simulink model "adaptiveObs"  (R2012b)
settings: Solver=ode45  StartTime=0.0  StopTime=TStop  MaxStep=Ts  RelTol=10e-5
values from neighbouring files (symbols this model uses):
  A = [-5 1; -10 0]    [adaptiveObsRun.m]
  a1hat0 = 3    [adaptiveObsRun.m]
  a2hat0 = 12    [adaptiveObsRun.m]
  B = [1;2]    [adaptiveObsRun.m]
  b1hat0 = 0.5    [adaptiveObsRun.m]
  b2hat0 = 1    [adaptiveObsRun.m]
  C = [1 0]    [adaptiveObsRun.m]
settings Model: Creator=sqn4594  LastModifiedBy=sqn4594
settings SolverCC: AlgebraicLoopSolver=LineSearch
settings DataIOCC: SignalLoggingSaveFormat=ModelDataLogs
settings DebuggingCC: MultiTaskDSMMsg=warning  MultiTaskCondExecSysMsg=none  StrictBusMsg=None
settings RTWCC: IncludeERTFirstTime=on
settings CodeAppCC: CustomSymbolStrType=$N$R$M_T  InternalIdentifier=Shortened

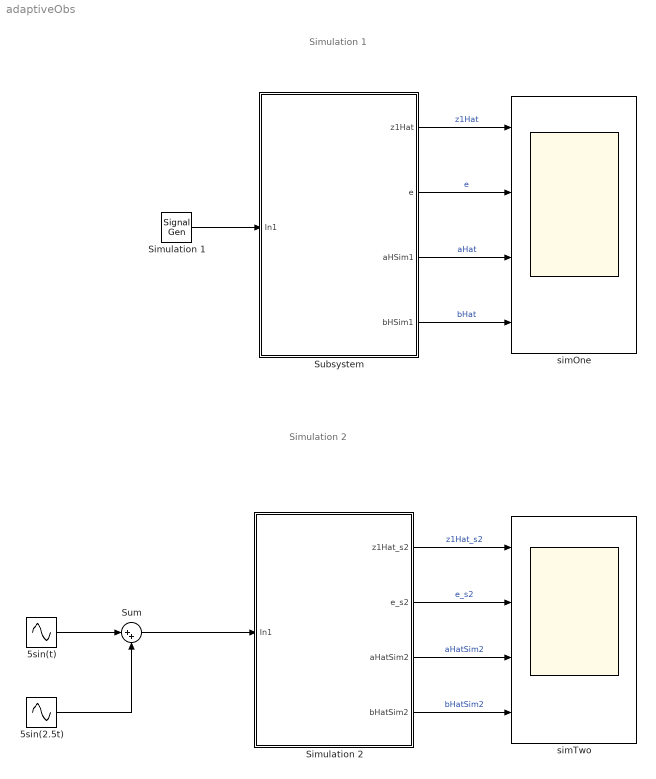
== system adaptiveObs ==
  note: Simulation 1
  note: Simulation 2
  5sin(2.5t) : Sin  Amplitude=5  Frequency=2.5  SampleTime=0
  5sin(t) : Sin  Amplitude=5  SampleTime=0
  Simulation 1 : SignalGenerator  WaveForm=square  Amplitude=5  Units=rad/sec
  Simulation 2 : Subsystem
  Subsystem : Subsystem
  Sum : Sum  Inputs=|++
  "simOne " : Scope  NumInputPorts=4
      settings: YMin=-5~-5~-5~-5  YMax=5~5~5~5  SaveName=simOne
  simTwo : Scope  NumInputPorts=4
      settings: YMin=-5~-5~-5~-5  YMax=5~5~5~5  SaveName=simTwo
  wires:
  5sin(t)/1 -> Sum/1
  5sin(2.5t)/1 -> Sum/2
  Simulation 1/1 -> Subsystem/1(In1)
  Sum/1 -> Simulation 2/1(In1)
  Subsystem/1(z1Hat) -> "simOne "/1  "z1Hat"
  Subsystem/2(e) -> "simOne "/2  "e"
  Subsystem/3(aHSim1) -> "simOne "/3  "aHat"
  Subsystem/4(bHSim1) -> "simOne "/4  "bHat"
  Simulation 2/1(z1Hat_s2) -> simTwo/1  "z1Hat_s2"
  Simulation 2/2(e_s2) -> simTwo/2  "e_s2"
  Simulation 2/3(aHatSim2) -> simTwo/3  "aHatSim2"
  Simulation 2/4(bHatSim2) -> simTwo/4  "bHatSim2"

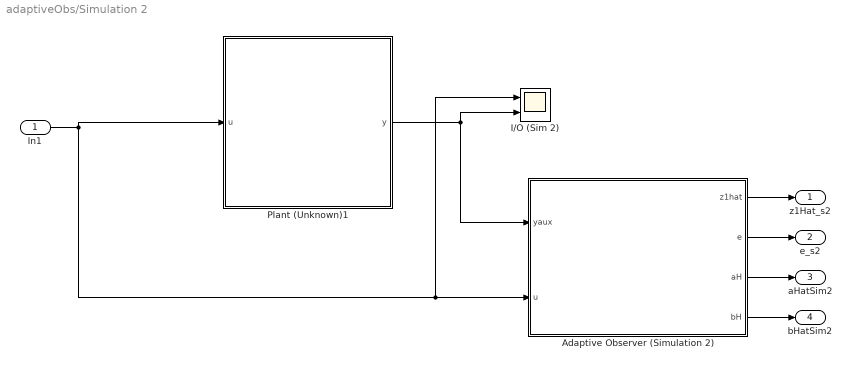
== system adaptiveObs/Simulation 2 ==
  In1 : Inport
  Adaptive Observer (Simulation 2) : Subsystem
  I/O (Sim 2) : Scope  NumInputPorts=2
      settings: YMin=-5~-5  YMax=5~5  SaveName=uy1
  Plant (Unknown)1 : Subsystem
  z1Hat_s2 : Outport
  e_s2 : Outport  Port=2
  aHatSim2 : Outport  Port=3
  bHatSim2 : Outport  Port=4
  wires:
  In1/1 -> Plant (Unknown)1/1(u), Adaptive Observer (Simulation 2)/2(u), I/O (Sim 2)/1
  Plant (Unknown)1/1(y) -> I/O (Sim 2)/2, Adaptive Observer (Simulation 2)/1(yaux)
  Adaptive Observer (Simulation 2)/1(z1hat) -> z1Hat_s2/1
  Adaptive Observer (Simulation 2)/2(e) -> e_s2/1
  Adaptive Observer (Simulation 2)/3(aH) -> aHatSim2/1
  Adaptive Observer (Simulation 2)/4(bH) -> bHatSim2/1

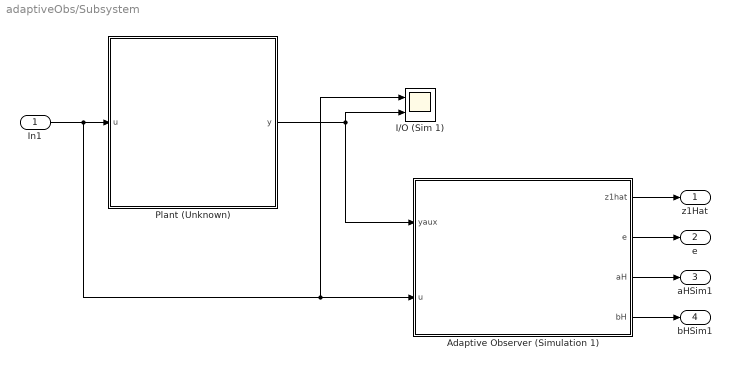
== system adaptiveObs/Subsystem ==
  In1 : Inport
  Adaptive Observer (Simulation 1) : Subsystem
  I/O (Sim 1) : Scope  NumInputPorts=2
      settings: YMin=-5~-5  YMax=5~5  SaveName=uy
  Plant (Unknown) : Subsystem
  z1Hat : Outport
  e : Outport  Port=2
  aHSim1 : Outport  Port=3
  bHSim1 : Outport  Port=4
  wires:
  Plant (Unknown)/1(y) -> Adaptive Observer (Simulation 1)/1(yaux), I/O (Sim 1)/2
  Adaptive Observer (Simulation 1)/1(z1hat) -> z1Hat/1
  In1/1 -> I/O (Sim 1)/1, Adaptive Observer (Simulation 1)/2(u), Plant (Unknown)/1(u)
  Adaptive Observer (Simulation 1)/2(e) -> e/1
  Adaptive Observer (Simulation 1)/3(aH) -> aHSim1/1
  Adaptive Observer (Simulation 1)/4(bH) -> bHSim1/1

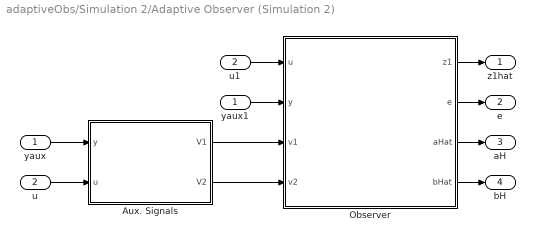
== system adaptiveObs/Simulation 2/Adaptive Observer (Simulation 2) ==
  yaux : Inport
  u : Inport  Port=2
  Aux. Signals : Subsystem
  Observer : Subsystem
      settings: MinAlgLoopOccurrences=on
  u1 : InportShadow  Port=2
  yaux1 : InportShadow
  z1hat : Outport
  e : Outport  Port=2
  aH : Outport  Port=3
  bH : Outport  Port=4
  wires:
  Observer/4(bHat) -> bH/1
  Observer/3(aHat) -> aH/1
  Observer/2(e) -> e/1
  Aux. Signals/2(V2) -> Observer/4(v2)
  Aux. Signals/1(V1) -> Observer/3(v1)
  Observer/1(z1) -> z1hat/1
  u1/1 -> Observer/1("u ")
  yaux1/1 -> Observer/2(y)
  u/1 -> Aux. Signals/2(u)
  yaux/1 -> Aux. Signals/1(y)

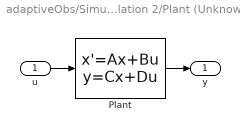
== system adaptiveObs/Simulation 2/Plant (Unknown)1 ==
  u : Inport
  Plant : StateSpace  A=A  B=B  C=C  D=0
  y : Outport
  wires:
  Plant/1 -> y/1
  u/1 -> Plant/1

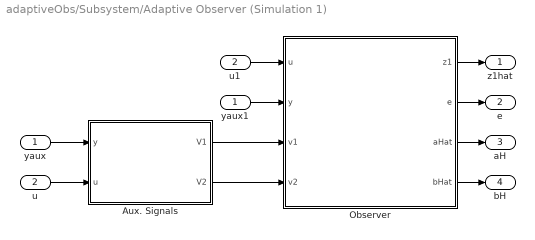
== system adaptiveObs/Subsystem/Adaptive Observer (Simulation 1) ==
  yaux : Inport
  u : Inport  Port=2
  Aux. Signals : Subsystem
  Observer : Subsystem
      settings: MinAlgLoopOccurrences=on
  u1 : InportShadow  Port=2
  yaux1 : InportShadow
  z1hat : Outport
  e : Outport  Port=2
  aH : Outport  Port=3
  bH : Outport  Port=4
  wires:
  yaux/1 -> Aux. Signals/1(y)
  u/1 -> Aux. Signals/2(u)
  yaux1/1 -> Observer/2(y)
  u1/1 -> Observer/1("u ")
  Observer/1(z1) -> z1hat/1
  Aux. Signals/1(V1) -> Observer/3(v1)
  Aux. Signals/2(V2) -> Observer/4(v2)
  Observer/2(e) -> e/1
  Observer/3(aHat) -> aH/1
  Observer/4(bHat) -> bH/1

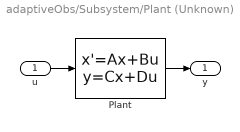
== system adaptiveObs/Subsystem/Plant (Unknown) ==
  u : Inport
  Plant : StateSpace  A=A  B=B  C=C  D=0
  y : Outport
  wires:
  u/1 -> Plant/1
  Plant/1 -> y/1

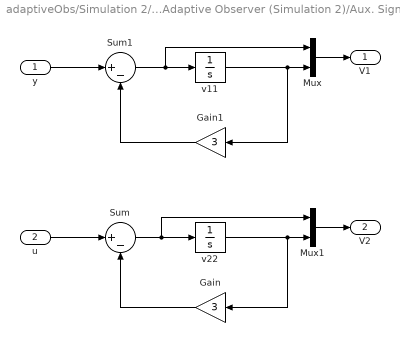
== system adaptiveObs/Simulation 2/Adaptive Observer (Simulation 2)/Aux. Signals ==
  y : Inport
  u : Inport  Port=2
  Gain : Gain  Gain=3
  Gain1 : Gain  Gain=3
  Mux : Mux  Inputs=2
  Mux1 : Mux  Inputs=2
  Sum : Sum  Inputs=|+-
  Sum1 : Sum  Inputs=|+-
  v11 : Integrator
  v22 : Integrator
  V1 : Outport
  V2 : Outport  Port=2
  wires:
  Mux1/1 -> V2/1
  Mux/1 -> V1/1
  v11/1 -> Mux/2, Gain1/1
  Gain1/1 -> Sum1/2
  y/1 -> Sum1/1
  Sum1/1 -> v11/1, Mux/1
  v22/1 -> Mux1/2, Gain/1
  Gain/1 -> Sum/2
  u/1 -> Sum/1
  Sum/1 -> v22/1, Mux1/1

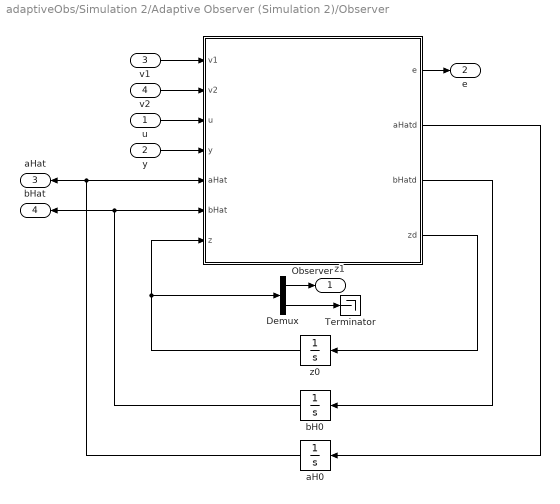
== system adaptiveObs/Simulation 2/Adaptive Observer (Simulation 2)/Observer ==
  "u " : Inport
  y : Inport  Port=2
  v1 : Inport  Port=3
  v2 : Inport  Port=4
  Demux : Demux  Outputs=2
  Observer : MATLAB Function  Priority=1
  Terminator : Terminator
  aH0 : Integrator  InitialCondition=[a1hat0;a2hat0]
  bH0 : Integrator  InitialCondition=[b1hat0;b2hat0]
  z0 : Integrator
  z1 : Outport
  e : Outport  Port=2
  aHat : Outport  Port=3
  bHat : Outport  Port=4
  wires:
  Demux/2 -> Terminator/1
  Demux/1 -> z1/1
  aH0/1 -> aHat/1, Observer/5(aHat)
  bH0/1 -> Observer/6(bHat), bHat/1
  Observer/1(e) -> e/1
  Observer/2(aHatd) -> aH0/1
  Observer/3(bHatd) -> bH0/1
  Observer/4(zd) -> z0/1
  y/1 -> Observer/4(y)
  "u "/1 -> Observer/3(u)
  v2/1 -> Observer/2(v2)
  v1/1 -> Observer/1(v1)
  z0/1 -> Observer/7(z), Demux/1

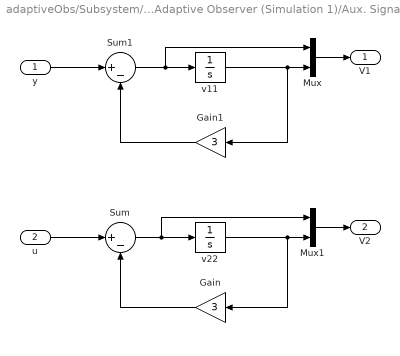
== system adaptiveObs/Subsystem/Adaptive Observer (Simulation 1)/Aux. Signals ==
  y : Inport
  u : Inport  Port=2
  Gain : Gain  Gain=3
  Gain1 : Gain  Gain=3
  Mux : Mux  Inputs=2
  Mux1 : Mux  Inputs=2
  Sum : Sum  Inputs=|+-
  Sum1 : Sum  Inputs=|+-
  v11 : Integrator
  v22 : Integrator
  V1 : Outport
  V2 : Outport  Port=2
  wires:
  Sum/1 -> Mux1/1, v22/1
  u/1 -> Sum/1
  Gain/1 -> Sum/2
  v22/1 -> Gain/1, Mux1/2
  Sum1/1 -> Mux/1, v11/1
  y/1 -> Sum1/1
  Gain1/1 -> Sum1/2
  v11/1 -> Gain1/1, Mux/2
  Mux/1 -> V1/1
  Mux1/1 -> V2/1

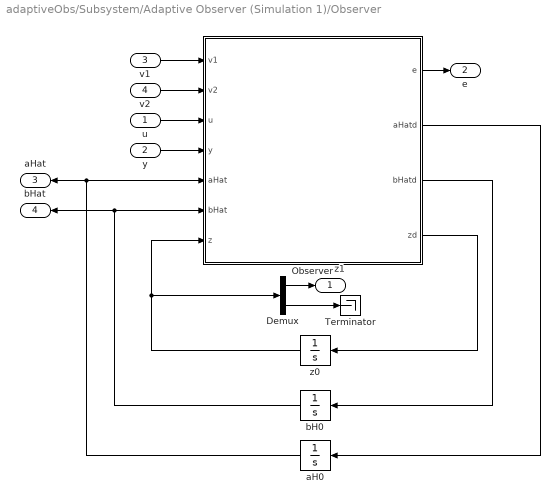
== system adaptiveObs/Subsystem/Adaptive Observer (Simulation 1)/Observer ==
  "u " : Inport
  y : Inport  Port=2
  v1 : Inport  Port=3
  v2 : Inport  Port=4
  Demux : Demux  Outputs=2
  Observer : MATLAB Function  Priority=1
  Terminator : Terminator
  aH0 : Integrator  InitialCondition=[a1hat0;a2hat0]
  bH0 : Integrator  InitialCondition=[b1hat0;b2hat0]
  z0 : Integrator
  z1 : Outport
  e : Outport  Port=2
  aHat : Outport  Port=3
  bHat : Outport  Port=4
  wires:
  z0/1 -> Demux/1, Observer/7(z)
  v1/1 -> Observer/1(v1)
  v2/1 -> Observer/2(v2)
  "u "/1 -> Observer/3(u)
  y/1 -> Observer/4(y)
  Observer/4(zd) -> z0/1
  Observer/3(bHatd) -> bH0/1
  Observer/2(aHatd) -> aH0/1
  Observer/1(e) -> e/1
  bH0/1 -> bHat/1, Observer/6(bHat)
  aH0/1 -> Observer/5(aHat), aHat/1
  Demux/1 -> z1/1
  Demux/2 -> Terminator/1

== matlab function adaptiveObs/Simulation 2/Adaptive Observer (Simulation 2)/Observer/Observer ==
  data: e output; aHatd output; bHatd output; zd output size=[2 1]; v1 input; v2 input; u input; y input; aHat input; bHat input; z input size=[2 1]
function [e,aHatd,bHatd,zd] = adObsSim2(v1,v2,u,y,aHat,bHat,z)
%#codegen
%% Consts
k1 = 6;
k2 = 8;
T1 = [140 0;0 75];
T2 = [5 0;0 7.8];
A2 = [0 -3;0 1];

%% Error
e = z(1)-y(1);

%% Adaptive 
aHatd = T1.*e*v1;
bHatd = -T2.*e*v2;

%% Observer 
Aobs = [-k1 1;-k2 0];
Aobs2= ([k1;k2]-aHat);
w = v1'*T1*A2*v1;
r = v2'*T2*A2*v2;
W = [0;w];
R = [0;r];
zd = Aobs*z+Aobs2*y+bHat*u-e.*(W+R);

== matlab function adaptiveObs/Subsystem/Adaptive Observer (Simulation 1)/Observer/Observer ==
  data: e output; aHatd output; bHatd output; zd output size=[2 1]; v1 input; v2 input; u input; y input; aHat input; bHat input; z input size=[2 1]
function [e,aHatd,bHatd,zd] = adObsSim1(v1,v2,u,y,aHat,bHat,z)
%#codegen
%% Consts
k1 = 6;
k2 = 8;
T1 = [23 0;0 3.8];
T2 = [2 0;0 0.4];
A2 = [0 -3;0 1];

%% Error
e = z(1)-y(1);

%% Adaptive 
aHatd = T1.*e*v1;
bHatd = -T2.*e*v2;

%% Observer 
Aobs = [-k1 1;-k2 0];
Aobs2= ([k1;k2]-aHat);
w = v1'*T1*A2*v1;
r = v2'*T2*A2*v2;
W = [0;w];
R = [0;r];
zd = Aobs*z+Aobs2*y+bHat*u-e.*(W+R);
